simulink model "week3_3"  (R2020b)
settings: Solver=VariableStepAuto  StartTime=0.0  StopTime=100  RelTol=1e-3
model workspace (MAT data in the model file):
  b1 = Simulink.Parameter
  b1.Value = 350
  b1.DataType = 'auto'
  b1.Dimensions = [1 1]
  b2 = Simulink.Parameter
  b2.Value = 15020
  b2.DataType = 'auto'
  b2.Dimensions = [1 1]
  k1 = Simulink.Parameter
  k1.Value = 80000
  k1.DataType = 'auto'
  k1.Dimensions = [1 1]
  k2 = Simulink.Parameter
  k2.Value = 500000
  k2.DataType = 'auto'
  k2.Dimensions = [1 1]
  m1 = Simulink.Parameter
  m1.Value = 2500
  m1.DataType = 'auto'
  m1.Dimensions = [1 1]
  m2 = Simulink.Parameter
  m2.Value = 320
  m2.DataType = 'auto'
  m2.Dimensions = [1 1]
settings Model: OrderedModelArguments=off  Creator=Lenovo  LastModifiedBy=Lenovo

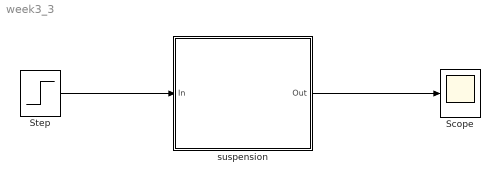
== system week3_3 ==
  Scope : Scope
  Step : Step  SampleTime=0
  suspension : Subsystem
  wires:
  Step/1 -> suspension/1(In)
  suspension/1(Out) -> Scope/1

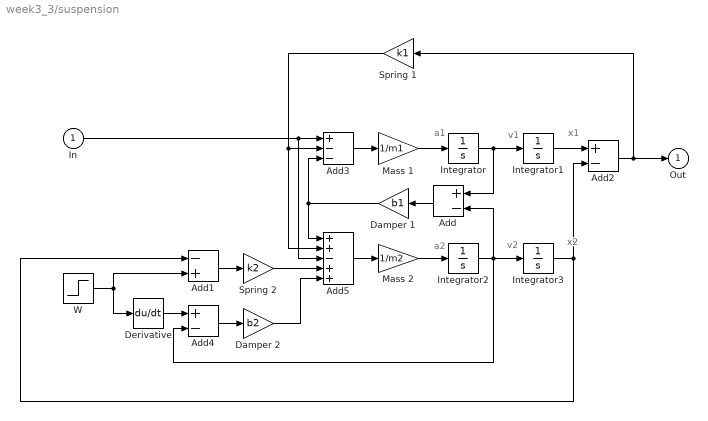
== system week3_3/suspension ==
  note: v1
  note: x1
  note: a2
  note: a1
  note: v2
  note: x2
  In : Inport
  Add : Sum  Inputs=+-
  Add1 : Sum  Inputs=-+
  Add2 : Sum  Inputs=+-
  Add3 : Sum  Inputs=+--
  Add4 : Sum  Inputs=+-
  Add5 : Sum  Inputs=++-++
  Damper 1 : Gain  Gain=b1
  Damper 2 : Gain  Gain=b2
  Derivative : Derivative
  Integrator{,1..3} (4 alike) : Integrator
  Mass 1 : Gain  Gain=1/m1
  Mass 2 : Gain  Gain=1/m2
  Spring 1 : Gain  Gain=k1
  Spring 2 : Gain  Gain=k2
  W : Step  Time=0  After=0
  Out : Outport  InitialOutput=0
  wires:
  Damper 1/1 -> Add3/3, Add5/1
  Spring 1/1 -> Add5/2, Add3/2
  Add/1 -> Damper 1/1
  Add2/1 -> Out/1, Spring 1/1
  Derivative/1 -> Add4/1
  Spring 2/1 -> Add5/4
  Integrator3/1 -> Add2/2, Add1/1
  In/1 -> Add5/3, Add3/1
  Integrator/1 -> Add/1, Integrator1/1
  Add5/1 -> Mass 2/1
  W/1 -> Derivative/1, Add1/2
  Integrator2/1 -> Add/2, Add4/2, Integrator3/1
  Mass 1/1 -> Integrator/1
  Mass 2/1 -> Integrator2/1
  Add4/1 -> Damper 2/1
  Integrator1/1 -> Add2/1
  Damper 2/1 -> Add5/5
  Add3/1 -> Mass 1/1
  Add1/1 -> Spring 2/1
